simulink model "Motor_PID_Control_wNL"  (R2025b)
settings: Solver=ode45  StartTime=0.0  StopTime=2  RelTol=1e-3
PreLoadFcn:
  | Kp=100;
  | Ki=200;
  | Kd=10;
InitFcn:
  | J = 0.01;
  | b = 0.1;
  | K = 0.01;
  | R = 1;
  | L = 0.5;
settings Model: Creator=sansh  LastModifiedBy=sjawahar
settings SolverCC: AlgebraicLoopSolver=TrustRegion
settings DataIOCC: ReturnWorkspaceOutputs=off
settings DebuggingCC: UnconnectedInputMsg=warning  UnconnectedOutputMsg=warning  UnconnectedLineMsg=warning  ArithmeticOperatorsInVariantConditions=warning
settings ModelReferenceCC: EnableRefExpFcnMdlSchedulingChecks=on
settings SFSimCC: SimUseLocalCustomCode=off  CustomCodeUndefinedFunction=UseInterfaceOnly
settings RTWCC: RTWUseLocalCustomCode=off  GPUComputeCapability=3.5
settings CodeAppCC: StateflowObjectComments=on

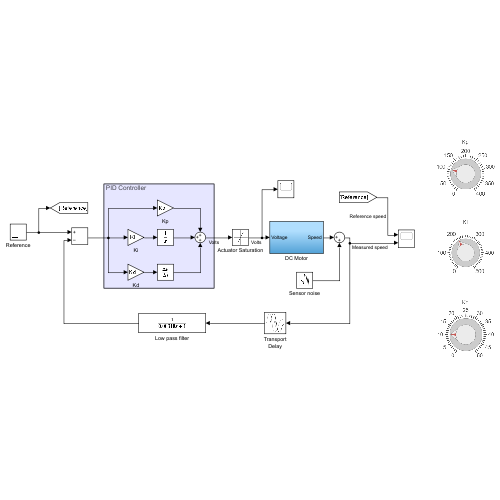
[thumbnail: Simulink's stored preview of the top-level diagram]
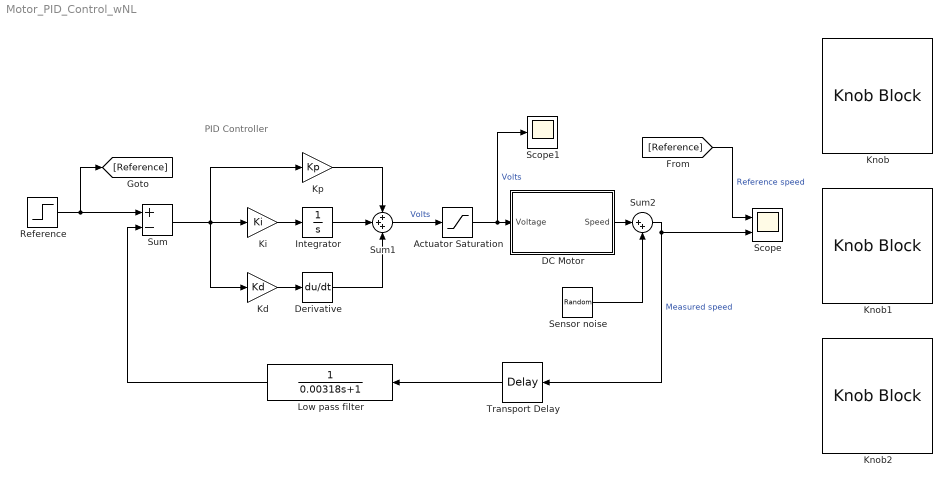
== system Motor_PID_Control_wNL ==
  note: PID Controller
  Actuator Saturation : Saturate  UpperLimit=48  LowerLimit=-48
  DC Motor : Subsystem
  Derivative : Derivative
  Integrator : Integrator
  Kd : Gain  Gain=Kd
  Ki : Gain  Gain=Ki
  Knob : KnobBlock  ScaleMax=400
  Knob1 : KnobBlock  ScaleMax=500
  Knob2 : KnobBlock  ScaleMax=50
  Kp : Gain  Gain=Kp
  Low pass filter : TransferFcn  Denominator=[0.00318 1]
  Reference : Step  Time=0  SampleTime=0
  Scope : Scope  NumInputPorts=2
      settings: ActiveDisplayYMinimum=-0.1653257876911669  ActiveDisplayYMaximum=1.3894435456865457
  Scope1 : Scope
      settings: ActiveDisplayYMinimum=-60  ActiveDisplayYMaximum=60
  Sensor noise : RandomNumber  Variance=0.0001  SampleTime=0.001
  Sum : Sum  Inputs=+-
  Sum1 : Sum  Inputs=+++
  Sum2 : Sum  Inputs=|++
  Transport Delay : TransportDelay  DelayTime=0.05
  wires:
  Reference/1 -> [Reference], Sum/1
  DC Motor/1(Speed) -> Sum2/1
  Sum1/1 -> Actuator Saturation/1  "Volts"
  Kp/1 -> Sum1/1
  Sum/1 -> Ki/1, Kd/1, Kp/1
  Integrator/1 -> Sum1/2
  Kd/1 -> Derivative/1
  Derivative/1 -> Sum1/3
  Ki/1 -> Integrator/1
  Actuator Saturation/1 -> Scope1/1, DC Motor/1(Voltage)  "Volts"
  Transport Delay/1 -> Low pass filter/1
  Sensor noise/1 -> Sum2/2
  Sum2/1 -> Transport Delay/1, Scope/2  "Measured speed"
  Low pass filter/1 -> Sum/2
  [Reference] -> Scope/1  "Reference speed"

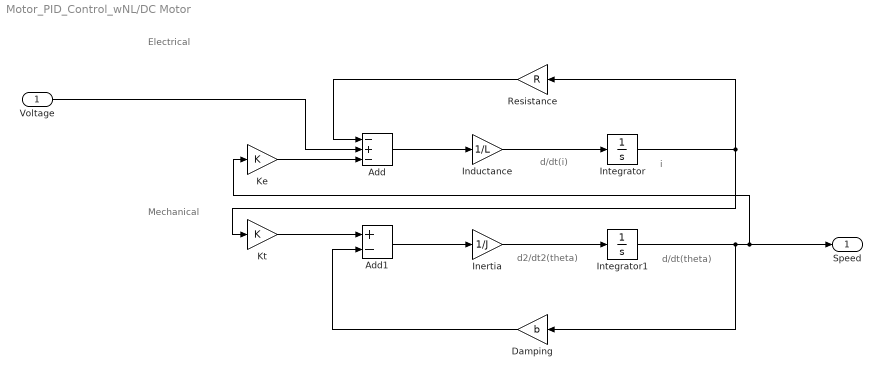
== system Motor_PID_Control_wNL/DC Motor ==
  note: Electrical
  note: Mechanical
  note: i
  note: d/dt(i)
  note: d/dt(theta)
  note: d2/dt2(theta)
  Voltage : Inport
  Add : Sum  Inputs=-+-
  Add1 : Sum  Inputs=+-
  Damping : Gain  Gain=b
  Inductance : Gain  Gain=1/L
  Inertia : Gain  Gain=1/J
  Integrator : Integrator
  Integrator1 : Integrator
  Ke : Gain  Gain=K
  Kt : Gain  Gain=K
  Resistance : Gain  Gain=R
  Speed : Outport
  wires:
  Inductance/1 -> Integrator/1
  Integrator1/1 -> Damping/1, Speed/1, Ke/1
  Inertia/1 -> Integrator1/1
  Integrator/1 -> Resistance/1, Kt/1
  Kt/1 -> Add1/1
  Voltage/1 -> Add/2
  Resistance/1 -> Add/1
  Damping/1 -> Add1/2
  Ke/1 -> Add/3
  Add/1 -> Inductance/1
  Add1/1 -> Inertia/1
